simulink model "ex01_simul"  (R2023a)
settings: Solver=VariableStepAuto  StartTime=0.0  StopTime=8  MaxStep=1e-3  RelTol=1e-3
values from neighbouring files (symbols this model uses):
  a = -7    [ex01.m]
  v1 = 25    [ex01.m]
settings Model: Creator=239026  LastModifiedBy=239026

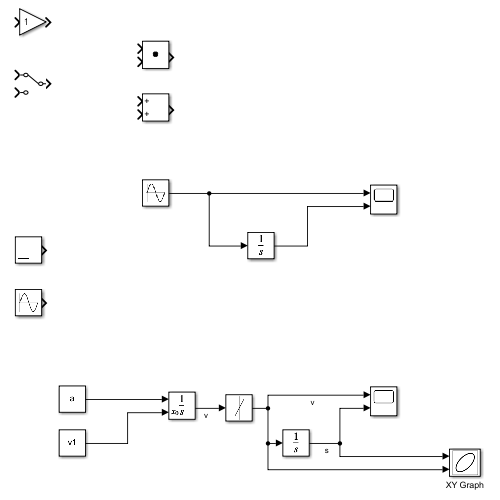
[thumbnail: Simulink's stored preview of the top-level diagram]
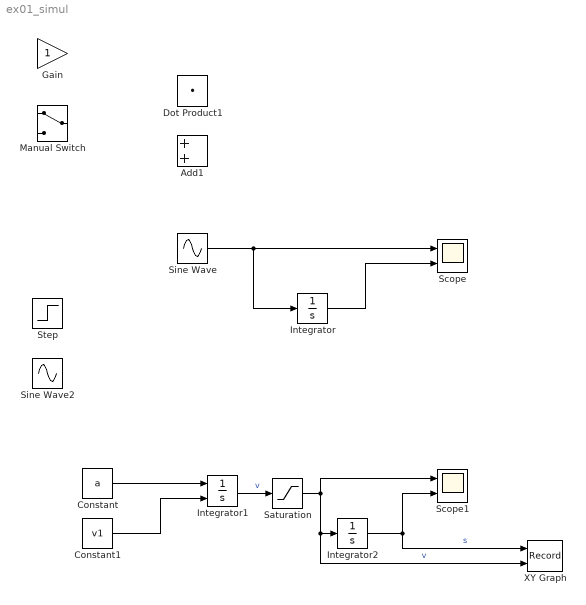
== system ex01_simul ==
  Add1 : Sum
  Constant : Constant  Value=a
  Constant1 : Constant  Value=v1
  Dot Product1 : DotProduct  OutDataTypeStr=Inherit: Inherit via internal rule
  Gain : Gain
  Integrator : Integrator
  Integrator1 : Integrator  InitialConditionSource=external
  Integrator2 : Integrator
  Manual Switch : ManualSwitch
  Saturation : Saturate  UpperLimit=Inf  LowerLimit=0
  Scope : Scope  NumInputPorts=2
  Scope1 : Scope  NumInputPorts=2
  Sine Wave : Sin  SampleTime=0
  Sine Wave2 : Sin  Frequency=2  Phase=1  SampleTime=0
  Step : Step  SampleTime=0
  XY Graph : Record  FileSettingsInternal="{\"entries\":[{\"content\":{\"excelSettings\":{\"content\":{},\"type\":\"Streamout.ExcelSettings\"}},\"type\":\"Streamout.FileSettingStorage\",\"uuid\":\"\"}],\"packageUris\":[\"http:\\/\\/schema.mathworks.com\\/mf0\\/streamout_blocks\\/R2020a\"],\"version\":\"1.0\"}"  Layout=[1 1]  SignalsInternal="{\"entries\":[{\"content\":{\"signals\":[{\"content\":{\"blockPath\":[],\"dimensions\":[1],\"domain\":\"\",\"lineColor\":\"#a2142f\",\"plots\":[1],\"port\":1,\"sid\":[\"\"],\"signalID\":21,\"signalName\":\"s\"},\"type\":\"RecordBlkView.Signal\",\"uuid\":\"\"},{\"content\":{\"blockPath\":[],\"dimensions\":[1],\"domain\":\"\",\"lineColor\":\"#139fff\",\"plots\":[1],\"port\":2,\"sid\":[\"\"],\"signalID\":25,\"signalName\":\"Saturation\"},\"type\":\"RecordBlkView.Signal\",\"uuid\":\"\"}]},\"type\":\"RecordBlkView.InputSignals\",\"uuid\":\"\"}],\"packageUris\":[\"http:\\/\\/schema.mathworks.com\\/mf0\\/streamout_blocks\\/R2020a\"],\"version\":\"1.0\"}"  VisualizationBindings="{\"xyplotplugin\":{\"info\":[{\"series\":[{\"bindingParametersList\":[{\"parameter\":\"X-Axis\",\"signalID\":21,\"signalName\":\"s\"},{\"parameter\":\"Y-Axis\",\"signalID\":25,\"signalName\":\"Saturation\"}],\"seriesID\":52408}],\"subplotID\":1}]}}"  CompatibilityTag=XY
  wires:
  Sine Wave/1 -> Integrator/1, Scope/1
  Integrator/1 -> Scope/2
  Constant/1 -> Integrator1/1
  Constant1/1 -> Integrator1/2
  Integrator1/1 -> Saturation/1  "v"
  Integrator2/1 -> Scope1/2, XY Graph/1  "s"
  Saturation/1 -> Integrator2/1, XY Graph/2, Scope1/1  "v"
